simulink model "ADS_model_2018"  (R2018a)
settings: Solver=FixedStepDiscrete  StartTime=0.0  StopTime=20  FixedStep=1/10  RelTol=1e-3
libraries: sldrtlib x1
settings Model: Creator=Admin  LastModifiedBy=Martin Dodek

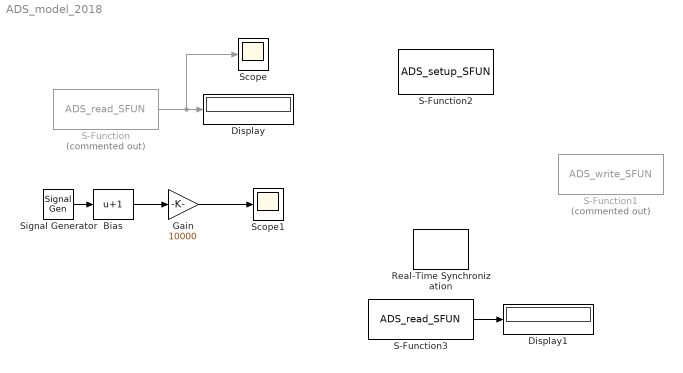
== system ADS_model_2018 ==
  Bias : Bias  Bias=1
  Display : Display
  Display1 : Display
  Gain : Gain  Gain=10000
  Real-Time Synchronization : sldrtlib/Real-Time Synchronization  SampleTime=0.1  MaxMissedTicks=10  ShowMissedTicks=off  YieldWhenWaiting=off
  S-Function : S-Function  Commented=on  FunctionName=ADS_read_SFUN  SFunctionDeploymentMode=off  EnableBusSupport=off
  S-Function1 : S-Function  Commented=on  FunctionName=ADS_write_SFUN  Parameters=[10, 3, 1, 138, 3, 1],'GVL.ventilator',4  SFunctionDeploymentMode=off  EnableBusSupport=off
  S-Function2 : S-Function  FunctionName=ADS_setup_SFUN  SFunctionDeploymentMode=off  EnableBusSupport=off
  S-Function3 : S-Function  FunctionName=ADS_read_SFUN  Parameters=[10, 3, 1, 138, 3, 1],'GVL.snimac1',4  SFunctionDeploymentMode=off  EnableBusSupport=off
  Scope : Scope
  Scope1 : Scope
  Signal Generator : SignalGenerator  Units=rad/sec
  wires:
  S-Function/1 -> Scope/1, Display/1
  Signal Generator/1 -> Bias/1
  Bias/1 -> Gain/1
  Gain/1 -> Scope1/1
  S-Function3/1 -> Display1/1
